simulink model "gmsk_tx_rx_tr"  (Simulink 7.9)
settings: Solver=FixedStepDiscrete  SolverMode=SingleTasking  StartTime=0.0  StopTime=1e2  RelTol=1e-3
undefined symbols (not defined in the file or in its folder): addr, gaussfir, get, gmsk_syn_params, N, sin_lut_length
libraries: shlslibv1 x67, commchan3 x1, commrandsrc2 x1, dsparch4 x1, commsink2 x1, commseqgen2 x1, commutil2 x1, dspsigops x1
settings Model: synDspstartup=OK  Creator=sszilvasi  LastModifiedBy=sszilvasi
settings DataIOCC: SaveOutput=off  SignalLogging=off  SaveTime=off
settings OptimizationCC: InlineParams=on
settings DebuggingCC: AlgebraicLoopMsg=error  InheritedTsInSrcMsg=none

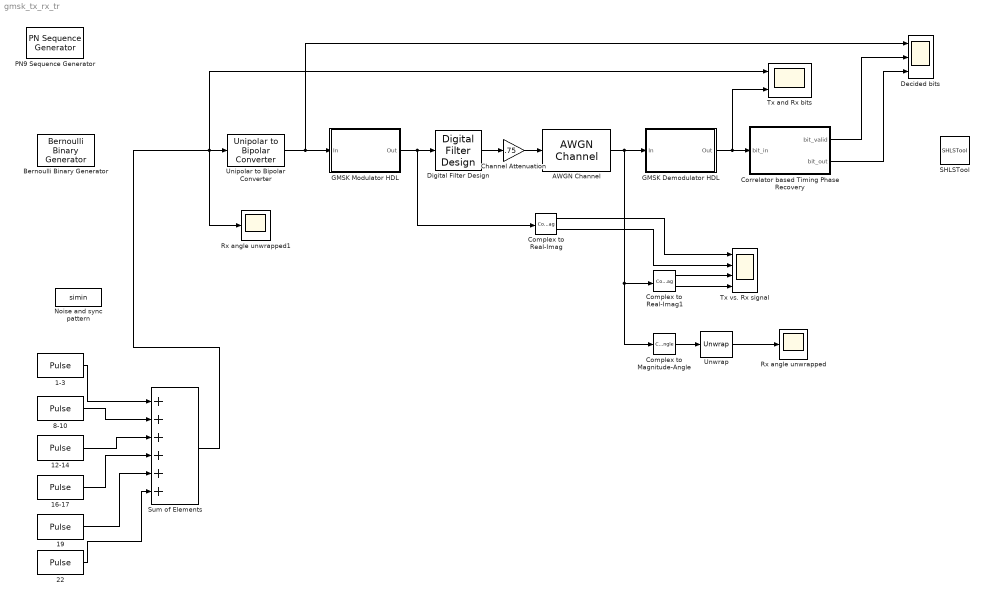
== system gmsk_tx_rx_tr ==
  1-3 : DiscretePulseGenerator  Period=100  PulseWidth=3  PhaseDelay=51
  12-14 : DiscretePulseGenerator  Period=100  PulseWidth=3  PhaseDelay=62
  16-17 : DiscretePulseGenerator  Period=100  PulseWidth=2  PhaseDelay=66
  19 : DiscretePulseGenerator  Period=100  PhaseDelay=69
  22 : DiscretePulseGenerator  Period=100  PhaseDelay=72
  8-10 : DiscretePulseGenerator  Period=100  PulseWidth=3  PhaseDelay=58
  AWGN Channel : commchan3/AWGN Channel  InputProcessing=Columns as channels (frame based)  seed=67  noiseMode="Signal to noise ratio  (Eb/No)"  EbNodB=25  EsNodB=10  SNRdB=10  bitsPerSym=1  Ps=1  Tsym=1  variance=1
  Bernoulli Binary Generator : commrandsrc2/Bernoulli Binary Generator  P=0.5  seed=61  Ts=1  frameBased=off  sampPerFrame=1  orient=off  outDataType=double
  Channel Attenuation : Gain  Gain=.75
  Complex to Magnitude-Angle : ComplexToMagnitudeAngle  Output=Angle
  Complex to Real-Imag : ComplexToRealImag
  Complex to Real-Imag1 : ComplexToRealImag
  Correlator based Timing Phase Recovery : Subsystem  mask{sync_pattern=[0 1 1 1 0 0 0 0 1 1 1 0 1 1 1 0 1 1 0 1 0 0 1 0]}
      mask prompts: sync_pattern "Synchronization pattern"
      mask Display:
      | port_label('input',1,'In')
      | port_label('output',1,'Valid')
      | port_label('output',2,'Out')
  Decided bits : Scope  NumInputPorts=3
      settings: YMin=-5~-5~-5  YMax=5~5~5  SaveName=ScopeData4
  Digital Filter Design : dsparch4/Digital Filter Design  mwdsp_browser_bugfix_var=off
  GMSK Demodulator HDL : Subsystem
  GMSK Modulator HDL : Subsystem
  Noise and sync pattern : FromWorkspace  VariableName=simin  SampleTime=0
  PN9 Sequence Generator : commseqgen2/PN Sequence Generator  poly=[1 0 0 0 1 0 0 0 0 1]  ini_sta=1  outBitMaskSource=Dialog parameter  shift=0  outVarSiz=off  maxOutSizeMode=Dialog parameter  maxOutSize=[10 1]  Ts=1  frameBased=off  sampPerFrame=1  reset=off  bitPackedOutputs=off  outDataType=double  numPackedBits=8  bitPackDataSigned=off  bitPackedOutDType=double
  Rx angle unwrapped : Scope
      settings: SaveName=ScopeData6
  Rx angle unwrapped1 : Scope
      settings: SaveName=ScopeData9
  SHLSTool : shlslibv1/SHLSTool  synBlockType=tool  syn_dsp_mode=FPGA
  Sum of Elements : Sum  Inputs=++++++
  Tx and Rx bits : Scope  NumInputPorts=2
      settings: YMin=-5~-5  YMax=5~5  SaveName=ScopeData7
  Tx vs. Rx signal : Scope  NumInputPorts=4
      settings: YMin=-5~-5~-1.1~-5  YMax=5~5~1.2~5  SaveName=ScopeData5
  Unipolar to Bipolar Converter : commutil2/Unipolar to Bipolar Converter  M=2  polarity=Positive  dataType=Inherit via internal rule
  Unwrap : dspsigops/Unwrap  tol=pi  InputProcessing=Columns as channels (frame based)  running=off
  wires:
  GMSK Modulator HDL/1(Out) -> Complex to Real-Imag/1, Digital Filter Design/1
  AWGN Channel/1 -> GMSK Demodulator HDL/1(In), Complex to Real-Imag1/1, Complex to Magnitude-Angle/1
  GMSK Demodulator HDL/1(Out) -> Correlator based Timing Phase Recovery/1(bit_in), Tx and Rx bits/2
  Correlator based Timing Phase Recovery/1(bit_valid) -> Decided bits/2
  Correlator based Timing Phase Recovery/2(bit_out) -> Decided bits/3
  Complex to Real-Imag/1 -> Tx vs. Rx signal/1
  Complex to Real-Imag/2 -> Tx vs. Rx signal/2
  Complex to Real-Imag1/1 -> Tx vs. Rx signal/3
  Complex to Real-Imag1/2 -> Tx vs. Rx signal/4
  Unwrap/1 -> Rx angle unwrapped/1
  Complex to Magnitude-Angle/1 -> Unwrap/1
  Sum of Elements/1 -> Unipolar to Bipolar Converter/1, Tx and Rx bits/1, Rx angle unwrapped1/1
  Unipolar to Bipolar Converter/1 -> GMSK Modulator HDL/1(In), Decided bits/1
  Channel Attenuation/1 -> AWGN Channel/1
  1-3/1 -> Sum of Elements/1
  8-10/1 -> Sum of Elements/2
  12-14/1 -> Sum of Elements/3
  16-17/1 -> Sum of Elements/4
  19/1 -> Sum of Elements/5
  22/1 -> Sum of Elements/6
  Digital Filter Design/1 -> Channel Attenuation/1

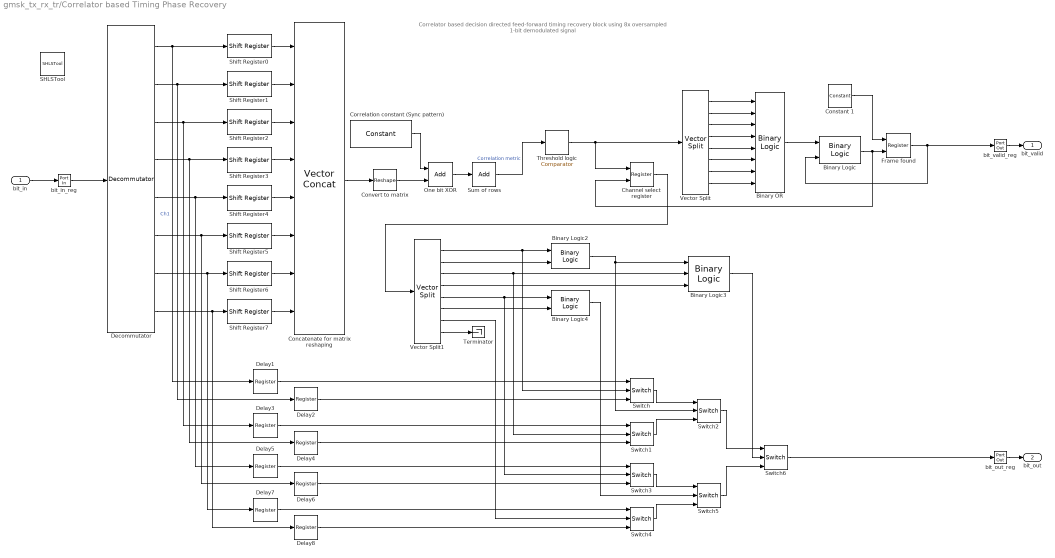
== system gmsk_tx_rx_tr/Correlator based Timing Phase Recovery ==
  note: Correlator based decision directed feed-forward timing recovery block
      | using 8x oversampled 1-bit demodulated signal
  bit_in : Inport
  Binary Logic : shlslibv1/Math Functions/Binary Logic  syn_binlog_exp=a&~b  synBlockType=primitive  synLatency=0  synBlockId=13
  Binary Logic2 : shlslibv1/Math Functions/Binary Logic  syn_binlog_exp=a|b  synBlockType=primitive  synLatency=0  synBlockId=13
  Binary Logic3 : shlslibv1/Math Functions/Binary Logic  syn_binlog_exp=a|b|c  synBlockType=primitive  synLatency=0  synBlockId=13
  Binary Logic4 : shlslibv1/Math Functions/Binary Logic  syn_binlog_exp=a|b  synBlockType=primitive  synLatency=0  synBlockId=13
  Binary OR : shlslibv1/Math Functions/Binary Logic  syn_binlog_exp=a|b|c|d|e|f|g|h  synBlockType=primitive  synLatency=0  synBlockId=13
  Channel select register : shlslibv1/Memories/Register  syn_delay_val=1  syn_rst_port=off  syn_en_port=on  synBlockType=custom  synLatency=1
  Concatenate for matrix reshaping : shlslibv1/Signal Operations/Vector Concat  syn_in_nb=8  syn_out_f=Full Precision  syn_out_wl=16  syn_out_fl=8  syn_out_dt=signed  synBlockType=primitive  synLatency=0  synBlockId=19
  Constant 1 : shlslibv1/Sources/Constant  syn_cst_val=1  syn_cst_fl=0  syn_cst_dt=unsigned  syn_cst_rnd=on  syn_cst_st=-1  synBlockType=primitive  synLatency=0  synBlockId=15
  Convert to matrix : shlslibv1/Signal Operations/Reshape  syn_op_dim_type=Specify  syn_op_dim=[length(sync_pattern) 8]  syn_ip_order=Row First  syn_op_order=Column First  syn_inh_port=off  synBlockType=primitive  synLatency=0  synBlockId=158
  Correlation constant (Sync pattern) : shlslibv1/Sources/Constant  syn_cst_val=fliplr([sync_pattern])'*ones(1,8)  syn_cst_fl=0  syn_cst_dt=unsigned  syn_cst_rnd=on  syn_cst_st=-1  synBlockType=primitive  synLatency=0  synBlockId=15
  Decommutator : shlslibv1/Signal Operations/Decommutator  syn_outport_nb=8  syn_outport_vec=off  synBlockType=custom  synLatency=1
  Delay{1..8} (8 alike) : shlslibv1/Memories/Register  syn_delay_val=1  syn_rst_port=off  syn_en_port=off  synBlockType=custom  synLatency=1
  Frame found : shlslibv1/Memories/Register  syn_delay_val=1  syn_rst_port=off  syn_en_port=on  synBlockType=custom  synLatency=1
  One bit XOR : shlslibv1/Math Functions/Add  syn_add_opr=++  syn_out_f=Specify  syn_out_wl=1  syn_out_fl=0  syn_out_dt=unsigned  syn_out_sat=off  syn_out_rnd=Floor (Truncate)  synBlockType=primitive  synLatency=0  synBlockId=96  syn_sum_of_rows=off
  SHLSTool : shlslibv1/SHLSTool  synBlockType=tool  syn_dsp_mode=FPGA
  Shift Register{0..7} (8 alike) : shlslibv1/Memories/Shift Register  syn_shift_dynamic=off  syn_shift_vec=[0:length(sync_pattern)-1]  syn_shift_val=16  syn_vect_out=Merge to vector  syn_rst_val=All zeros  syn_rst_vec=0  syn_rst_port=off  syn_en_port=off  synBlockType=primitive  synLatency=(addr+1)  synBlockId=93
  Sum of rows : shlslibv1/Math Functions/Add  syn_add_opr=+  syn_out_f=Specify  syn_out_wl=5  syn_out_fl=0  syn_out_dt=unsigned  syn_out_sat=off  syn_out_rnd=Floor (Truncate)  synBlockType=primitive  synLatency=0  synBlockId=96  syn_sum_of_rows=on
  Switch{,1..6} (7 alike) : shlslibv1/Signal Operations/Switch  switchCriteria=u2 > Threshold  switchThresh=0  synBlockType=custom  synLatency=0
  Terminator : Terminator
  Threshold logic : shlslibv1/Math Functions/Comparator  syn_comp_opr=a==b  syn_comp_const=on  syn_comp_val=0  synBlockType=primitive  synLatency=0  synBlockId=14
  Vector Split : shlslibv1/Signal Operations/Vector Split  syn_out_nb=8  synBlockType=primitive  synLatency=0  synBlockId=20
  Vector Split1 : shlslibv1/Signal Operations/Vector Split  syn_out_nb=8  synBlockType=primitive  synLatency=0  synBlockId=20
  bit_in_reg : shlslibv1/Ports & Subsystems/Port In  syn_out_wl=1  syn_out_fl=0  syn_out_dt=unsigned  syn_out_st=-1  syn_capture=off  syn_register=on  syn_out_sat=off  syn_out_rnd=on  synBlockType=port  synLatency=1  synBlockId=0
  bit_out_reg : shlslibv1/Ports & Subsystems/Port Out  syn_capture=off  syn_register=on  synBlockType=port  synLatency=1  synBlockId=1
  bit_valid_reg : shlslibv1/Ports & Subsystems/Port Out  syn_capture=off  syn_register=on  synBlockType=port  synLatency=1  synBlockId=1
  bit_valid : Outport
  bit_out : Outport  Port=2
  wires:
  Decommutator/1 -> Shift Register0/1, Delay1/1  "Ch1"
  Decommutator/2 -> Shift Register1/1, Delay2/1
  Decommutator/3 -> Shift Register2/1, Delay3/1
  Decommutator/4 -> Shift Register3/1, Delay4/1
  Shift Register0/1 -> Concatenate for matrix reshaping/1
  Shift Register1/1 -> Concatenate for matrix reshaping/2
  Shift Register2/1 -> Concatenate for matrix reshaping/3
  Shift Register3/1 -> Concatenate for matrix reshaping/4
  Sum of rows/1 -> Threshold logic/1  "Correlation metric"
  One bit XOR/1 -> Sum of rows/1
  Concatenate for matrix reshaping/1 -> Convert to matrix/1
  Vector Split/1 -> Binary OR/1
  Vector Split/2 -> Binary OR/2
  Vector Split/3 -> Binary OR/3
  Vector Split/4 -> Binary OR/4
  Switch/1 -> Switch2/1
  Switch1/1 -> Switch2/3
  Binary OR/1 -> Binary Logic/1
  Frame found/1 -> Binary Logic/2, bit_valid_reg/1
  Binary Logic/1 -> Frame found/2, Channel select register/2
  Constant 1/1 -> Frame found/1
  Vector Split1/1 -> Switch/2, Binary Logic2/1
  Vector Split1/3 -> Switch1/2, Binary Logic3/2
  Binary Logic2/1 -> Switch2/2, Binary Logic3/1
  Vector Split1/2 -> Binary Logic2/2
  Threshold logic/1 -> Vector Split/1, Channel select register/1
  Correlation constant (Sync pattern)/1 -> One bit XOR/1
  Decommutator/5 -> Shift Register4/1, Delay5/1
  Decommutator/6 -> Shift Register5/1, Delay6/1
  Decommutator/7 -> Shift Register6/1, Delay7/1
  Decommutator/8 -> Shift Register7/1, Delay8/1
  Shift Register4/1 -> Concatenate for matrix reshaping/5
  Shift Register5/1 -> Concatenate for matrix reshaping/6
  Shift Register6/1 -> Concatenate for matrix reshaping/7
  Shift Register7/1 -> Concatenate for matrix reshaping/8
  Vector Split/5 -> Binary OR/5
  Vector Split/6 -> Binary OR/6
  Vector Split/7 -> Binary OR/7
  Vector Split/8 -> Binary OR/8
  Switch3/1 -> Switch5/1
  Switch4/1 -> Switch5/3
  Switch5/1 -> Switch6/3
  Switch2/1 -> Switch6/1
  Switch6/1 -> bit_out_reg/1
  Vector Split1/5 -> Switch3/2, Binary Logic4/1
  Vector Split1/7 -> Switch4/2
  Vector Split1/6 -> Binary Logic4/2
  Binary Logic4/1 -> Switch5/2
  Vector Split1/4 -> Binary Logic3/3
  Binary Logic3/1 -> Switch6/2
  Convert to matrix/1 -> One bit XOR/2
  bit_in_reg/1 -> Decommutator/1
  bit_in/1 -> bit_in_reg/1
  bit_valid_reg/1 -> bit_valid/1
  bit_out_reg/1 -> bit_out/1
  Vector Split1/8 -> Terminator/1
  Channel select register/1 -> Vector Split1/1
  Delay1/1 -> Switch/1
  Delay2/1 -> Switch/3
  Delay3/1 -> Switch1/1
  Delay4/1 -> Switch1/3
  Delay5/1 -> Switch3/1
  Delay6/1 -> Switch3/3
  Delay7/1 -> Switch4/1
  Delay8/1 -> Switch4/3

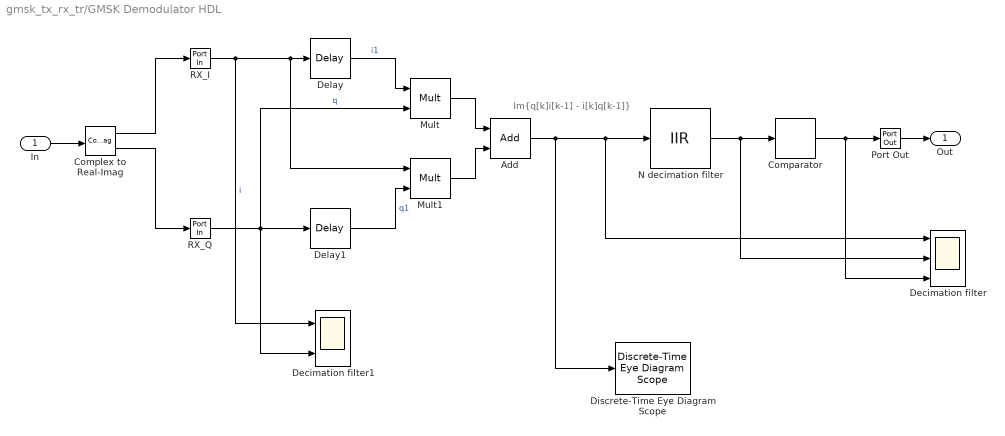
== system gmsk_tx_rx_tr/GMSK Demodulator HDL ==
  note: Im{q[k]i[k-1] - i[k]q[k-1]}
  In : Inport
  Add : shlslibv1/Math Functions/Add  syn_add_opr=+-  syn_out_f=Full Precision  syn_out_wl=2  syn_out_fl=0  syn_out_dt=signed  syn_out_sat=off  syn_out_rnd=Floor (Truncate)  synBlockType=primitive  synLatency=0  synBlockId=96  syn_sum_of_rows=off
  Comparator : shlslibv1/Math Functions/Comparator  syn_comp_opr=a>=b  syn_comp_const=on  syn_comp_val=0  synBlockType=primitive  synLatency=0  synBlockId=14
  Complex to Real-Imag : ComplexToRealImag
  Decimation filter : Scope  NumInputPorts=3
      settings: YMin=-5~-5~-5  YMax=5~5~5  SaveName=ScopeData2
  Decimation filter1 : Scope  NumInputPorts=2
      settings: YMin=-5~-5  YMax=5~5  SaveName=ScopeData8
  Delay : shlslibv1/Memories/Delay  syn_delay_val=1  synBlockType=primitive  synLatency=1  synBlockId=104
  Delay1 : shlslibv1/Memories/Delay  syn_delay_val=1  synBlockType=primitive  synLatency=1  synBlockId=104
  Discrete-Time Eye Diagram Scope : commsink2/Discrete-Time Eye Diagram Scope  Tag=EyeDiagram  sampPerSymb=8  offsetEye=0  symbPerTrace=2  numTraces=40  numNewFrames=40  LineStyles=-  LineColors=b  dupPoints=on  fading=on  render=on  AxisGrid=on  yMin=-0.16126880645752  yMax=0.148855781555176  inphaseLabel=In-phase Amplitude  quadratureLabel=Quadrature Amplitude  openScopeAtSimStart=off  dispDiagram=In-phase Only  FrameNumber=off  FigPos=get(0,'defaultfigureposition');  figTitle=Eye Diagram  block_type_=eye  numLinesMax=8
  Mult : shlslibv1/Math Functions/Mult  syn_out_f=Full Precision  syn_out_wl=16  syn_out_fl=8  syn_out_dt=signed  syn_out_sat=off  syn_out_rnd=Floor (Truncate)  synBlockType=primitive  synLatency=0  synBlockId=3  syn_opr_mode=1
  Mult1 : shlslibv1/Math Functions/Mult  syn_out_f=Full Precision  syn_out_wl=16  syn_out_fl=8  syn_out_dt=signed  syn_out_sat=off  syn_out_rnd=Floor (Truncate)  synBlockType=primitive  synLatency=0  synBlockId=3  syn_opr_mode=1
  N decimation filter : shlslibv1/Filtering/IIR  syn_coefb_vec=[1 zeros(1,N-2) -1]/N  syn_coefa_vec=[1 -1]  syn_coef_fl=8  syn_coef_rnd=on  syn_show_q=off  syn_out_f=Automatic  syn_out_wl=16  syn_out_fl=8  syn_out_dt=signed  syn_out_sat=off  syn_out_rnd=Floor (Truncate)  synBlockType=primitive  synLatency=0  synBlockId=83
  Port Out : shlslibv1/Ports & Subsystems/Port Out  syn_capture=off  syn_register=on  synBlockType=port  synLatency=1  synBlockId=1
  RX_I : shlslibv1/Ports & Subsystems/Port In  syn_out_wl=10  syn_out_fl=9  syn_out_dt=signed  syn_out_st=-1  syn_capture=off  syn_register=off  syn_out_sat=off  syn_out_rnd=off  synBlockType=port  synLatency=0  synBlockId=0
  RX_Q : shlslibv1/Ports & Subsystems/Port In  syn_out_wl=10  syn_out_fl=9  syn_out_dt=signed  syn_out_st=-1  syn_capture=off  syn_register=off  syn_out_sat=off  syn_out_rnd=off  synBlockType=port  synLatency=0  synBlockId=0
  Out : Outport
  wires:
  Complex to Real-Imag/1 -> RX_I/1
  Complex to Real-Imag/2 -> RX_Q/1
  RX_Q/1 -> Mult/2, Delay1/1, Decimation filter1/2  "q"
  RX_I/1 -> Delay/1, Mult1/1, Decimation filter1/1  "i"
  Delay/1 -> Mult/1  "i1"
  Delay1/1 -> Mult1/2  "q1"
  Mult/1 -> Add/1
  Mult1/1 -> Add/2
  Add/1 -> N decimation filter/1, Decimation filter/1, Discrete-Time Eye Diagram Scope/1
  In/1 -> Complex to Real-Imag/1
  N decimation filter/1 -> Decimation filter/2, Comparator/1
  Comparator/1 -> Decimation filter/3, Port Out/1
  Port Out/1 -> Out/1

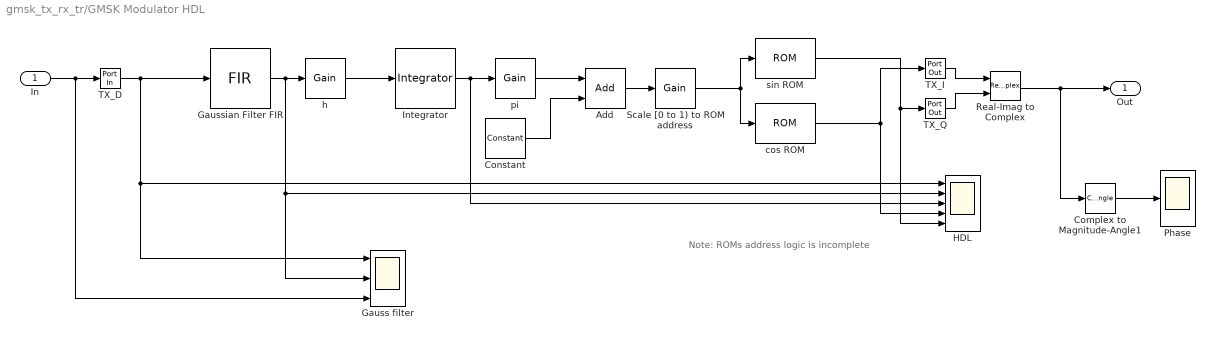
== system gmsk_tx_rx_tr/GMSK Modulator HDL ==
  note: Note: ROMs address logic is incomplete
  In : Inport
  Add : shlslibv1/Math Functions/Add  syn_add_opr=++  syn_out_f=Automatic  syn_out_wl=5  syn_out_fl=5  syn_out_dt=unsigned  syn_out_sat=off  syn_out_rnd=Floor (Truncate)  synBlockType=primitive  synLatency=0  synBlockId=96  syn_sum_of_rows=off
  Complex to Magnitude-Angle1 : ComplexToMagnitudeAngle  Output=Angle
  Constant : shlslibv1/Sources/Constant  syn_cst_val=.5  syn_cst_fl=1  syn_cst_dt=signed  syn_cst_rnd=on  syn_cst_st=-1  synBlockType=primitive  synLatency=0  synBlockId=15
  Gauss filter : Scope  NumInputPorts=3
      settings: YMin=-5~-5~-5  YMax=5~5~5
  Gaussian Filter FIR : shlslibv1/Filtering/FIR  syn_coef_vec=gaussfir(0.5,1,8)  syn_coef_fl=15  syn_coef_rnd=Nearest  syn_show_q=off  syn_dp_f=Automatic  syn_dp_wl=16  syn_dp_fl=8  syn_dp_sat=off  syn_dp_rnd=Floor (Truncate)  syn_out_f=Full Precision  syn_out_wl=16  syn_out_fl=8  syn_out_dt=signed  syn_out_sat=off  syn_out_rnd=Floor (Truncate)  syn_rst_port=off  syn_en_port=off  synBlockType=primitive  synLatency=0  synBlockId=80
  HDL : Scope  NumInputPorts=5
      settings: YMin=-5~-5~-5~-5~-5  YMax=5~5~5~5~5
  Integrator : shlslibv1/Filtering/Integrator  syn_pole_val=1  syn_feedback_fl=8  syn_out_f=Automatic  syn_out_wl=16  syn_out_fl=8  syn_out_dt=signed  syn_out_sat=off  syn_out_rnd=off  syn_rst_port=off  syn_en_port=off  synBlockType=custom  synLatency=0
  Phase : Scope
      settings: SaveName=ScopeData3
  Real-Imag to Complex : RealImagToComplex
  Scale [0 to 1) to ROM address : shlslibv1/Math Functions/Gain  syn_gain_val=sin_lut_length  syn_gain_fl=15  syn_gain_dt=signed  syn_gain_rnd=on  syn_out_f=Specify  syn_out_wl=6  syn_out_fl=0  syn_out_dt=unsigned  syn_out_sat=off  syn_out_rnd=Floor (Truncate)  synBlockType=primitive  synLatency=0  synBlockId=3  syn_opr_mode=0
  TX_D : shlslibv1/Ports & Subsystems/Port In  syn_out_wl=16  syn_out_fl=14  syn_out_dt=signed  syn_out_st=1/8  syn_capture=on  syn_register=off  syn_out_sat=off  syn_out_rnd=on  synBlockType=port  synLatency=0  synBlockId=0
  TX_I : shlslibv1/Ports & Subsystems/Port Out  syn_capture=off  syn_register=off  synBlockType=port  synLatency=0  synBlockId=1
  TX_Q : shlslibv1/Ports & Subsystems/Port Out  syn_capture=off  syn_register=off  synBlockType=port  synLatency=0  synBlockId=1
  cos ROM : shlslibv1/Memories/ROM  syn_rom_vec=cos(pi*2*[0:sin_lut_length-1]/sin_lut_length)  syn_out_wl=10  syn_out_fl=9  syn_out_dt=signed  syn_out_sat=on  syn_out_rnd=on  synBlockType=primitive  synLatency=1  synBlockId=62
  h : shlslibv1/Math Functions/Gain  syn_gain_val=1/4  syn_gain_fl=15  syn_gain_dt=signed  syn_gain_rnd=on  syn_out_f=Full Precision  syn_out_wl=16  syn_out_fl=8  syn_out_dt=signed  syn_out_sat=off  syn_out_rnd=Floor (Truncate)  synBlockType=primitive  synLatency=0  synBlockId=3  syn_opr_mode=0
  pi : shlslibv1/Math Functions/Gain  syn_gain_val=1/gmsk_syn_params.N  syn_gain_fl=15  syn_gain_dt=signed  syn_gain_rnd=on  syn_out_f=Full Precision  syn_out_wl=16  syn_out_fl=8  syn_out_dt=signed  syn_out_sat=off  syn_out_rnd=Floor (Truncate)  synBlockType=primitive  synLatency=0  synBlockId=3  syn_opr_mode=0
  sin ROM : shlslibv1/Memories/ROM  syn_rom_vec=sin(pi*2*[0:gmsk_syn_params.sin_lut_length-1]/gmsk_syn_params.sin_lut_length)  syn_out_wl=10  syn_out_fl=9  syn_out_dt=signed  syn_out_sat=on  syn_out_rnd=on  synBlockType=primitive  synLatency=1  synBlockId=62
  Out : Outport
  wires:
  Complex to Magnitude-Angle1/1 -> Phase/1
  In/1 -> TX_D/1, Gauss filter/3
  TX_D/1 -> HDL/1, Gauss filter/1, Gaussian Filter FIR/1
  Scale [0 to 1) to ROM address/1 -> sin ROM/1, cos ROM/1
  Constant/1 -> Add/2
  pi/1 -> Add/1
  Real-Imag to Complex/1 -> Complex to Magnitude-Angle1/1, Out/1
  sin ROM/1 -> HDL/5, TX_Q/1
  cos ROM/1 -> TX_I/1, HDL/4
  Add/1 -> Scale [0 to 1) to ROM address/1
  Integrator/1 -> pi/1, HDL/3
  h/1 -> Integrator/1
  TX_Q/1 -> Real-Imag to Complex/2
  TX_I/1 -> Real-Imag to Complex/1
  Gaussian Filter FIR/1 -> h/1, HDL/2, Gauss filter/2
